simulink model "main"  (R2023b)
settings: Solver=FixedStepAuto  StartTime=0.0  StopTime=T  FixedStep=dt  RelTol=1e-3
values from neighbouring files (symbols this model uses):
  ctrl_dt = 1e-4    (= 0.0001)    [main_slx.m]
  x = [0;0]    [main_slx.m]
settings Model: Creator=dding  LastModifiedBy=dding

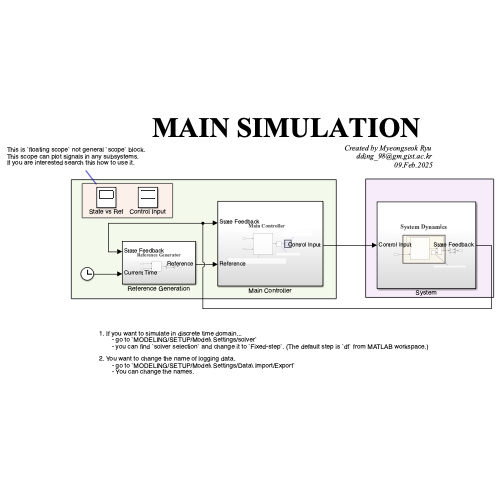
[thumbnail: Simulink's stored preview of the top-level diagram]
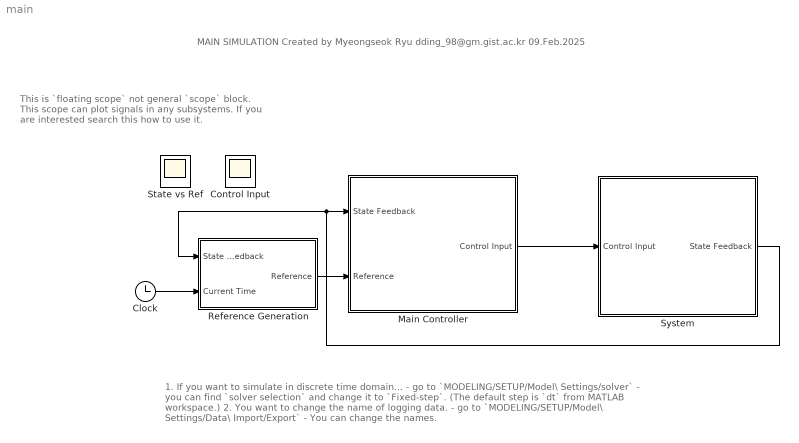
== system main ==
  note: 1. If you want to simulate in discrete time domain...
      | 	- go to `MODELING/SETUP/Model\ Settings/solver`
      | 	- you can find `solver selection` and change it to `Fixed-step`. (The default step is `dt` from MATLAB workspace.)
      |
      | 2. You want to change the name of logging data.
      | 	- go to `MODELING/SETUP/Model\ Settings/Data\ Import/Export`
      | 	- You can change the names.
  note: This is `floating scope` not general `scope` block.
      | This scope can plot signals in any subsystems.
      | If you are interested search this how to use it.
  note: MAIN SIMULATION
      | Created by Myeongseok Ryu
      | dding_98@gm.gist.ac.kr
      | 09.Feb.2025
  Clock : Clock
  Control Input : Scope
      settings: Floating=on
  Main Controller : Subsystem
  Reference Generation : Subsystem
  State vs Ref : Scope
      settings: Floating=on
  System : Subsystem
  wires:
  Clock/1 -> Reference Generation/2(Current Time)
  Reference Generation/1(Reference) -> Main Controller/2(Reference)
  Main Controller/1(Control Input) -> System/1(Control Input)
  System/1(State Feedback) -> Main Controller/1(State Feedback), Reference Generation/1(State Feedback)

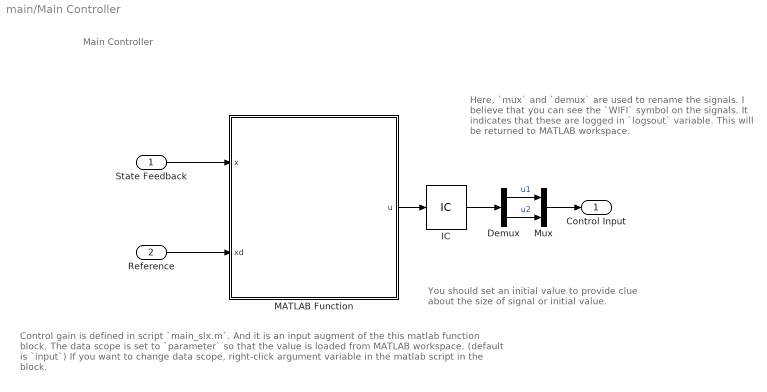
== system main/Main Controller ==
  note: Here, `mux` and `demux` are used to rename the signals.
      |
      | I believe that you can see the `WIFI` symbol on the signals.
      | It indicates that these are logged in `logsout` variable.
      | This will be returned to MATLAB workspace.
  note: You should set an initial value to provide clue about the size of signal or initial value.
  note: Control gain is defined in script `main_slx.m`.
      | And it is an input augment of the this matlab function block.
      | The data scope is set to `parameter` so that the value is loaded from MATLAB workspace. (default is `input`)
      | If you want to change data scope, right-click argument variable in the matlab script in the block.
  note: Main Controller
  State Feedback : Inport
  Reference : Inport  Port=2
  Demux : Demux  Outputs=2
  IC : InitialCondition  Value=u
  MATLAB Function : MATLAB Function  TreatAsAtomicUnit=on  SystemSampleTime=ctrl_dt
  Mux : Mux  Inputs=2
  Control Input : Outport
  wires:
  Reference/1 -> MATLAB Function/2(xd)
  MATLAB Function/1(u) -> IC/1
  State Feedback/1 -> MATLAB Function/1(x)
  Mux/1 -> Control Input/1
  Demux/1 -> Mux/1  "u1"
  Demux/2 -> Mux/2  "u2"
  IC/1 -> Demux/1

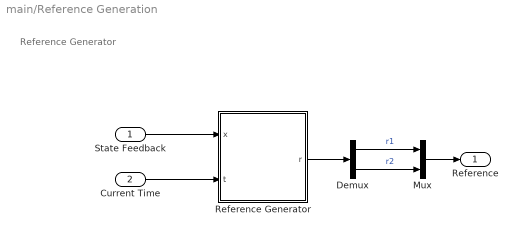
== system main/Reference Generation ==
  note: Reference Generator
  State Feedback : Inport
  Current Time : Inport  Port=2
  Demux : Demux  Outputs=2
  Mux : Mux  Inputs=2
  Reference Generator : MATLAB Function  TreatAsAtomicUnit=on
  Reference : Outport
  wires:
  State Feedback/1 -> Reference Generator/1(x)
  Reference Generator/1(r) -> Demux/1
  Current Time/1 -> Reference Generator/2(t)
  Mux/1 -> Reference/1
  Demux/1 -> Mux/1  "r1"
  Demux/2 -> Mux/2  "r2"

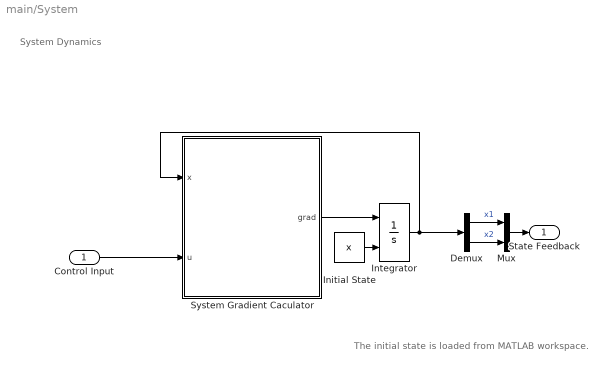
== system main/System ==
  note: The initial state is loaded from MATLAB workspace.
  note: System Dynamics
  Control Input : Inport
  Demux : Demux  Outputs=2
  Initial State : Constant  Value=x
  Integrator : Integrator  InitialConditionSource=external
  Mux : Mux  Inputs=2
  System Gradient Caculator : MATLAB Function  TreatAsAtomicUnit=on
  State Feedback : Outport
  wires:
  System Gradient Caculator/1(grad) -> Integrator/1
  Integrator/1 -> System Gradient Caculator/1(x), Demux/1
  Initial State/1 -> Integrator/2
  Mux/1 -> State Feedback/1
  Demux/1 -> Mux/1  "x1"
  Demux/2 -> Mux/2  "x2"
  Control Input/1 -> System Gradient Caculator/2(u)

== matlab function main/System/System Gradient Caculator ==
  data: x input; u input; grad output
function grad = fcn(x, u)
    A = [0 1; -2 -3];      % system matrix
    B = eye(2);            % input matrix

    grad = A*x + B*u;
end

== matlab function main/Reference Generation/Reference Generator ==
  data: x input; r output; t input
function r = fcn(x, t)

% Appetizer
r = [
    sin(t);
    cos(t);
];

== matlab function main/Main Controller/MATLAB Function ==
  data: x input; u output; xd input; K parameter
function u = fcn(x, xd, K)

u = -K*(x-xd);
